simulink model "Example_model"  (R2024b)
settings: Solver=VariableStepAuto  StartTime=0.0  StopTime=60  MaxStep=0.01  RelTol=1e-3
model workspace (MAT data in the model file):
  Sig = Simulink.Signal
  Sig.Dimensions = -1
  Sig.DimensionsMode = 'auto'
  Sig.Complexity = 'auto'
  Sig.SampleTime = -1
  Sig.SamplingMode = 'auto'
  Sig.DataType = 'auto'
  a0 = Simulink.Parameter
  a0.Value = 1
  a0.Complexity = 'real'
  a0.Dimensions = [1 1]
  a0.DataType = 'double'
  a1 = Simulink.Parameter
  a1.Value = 1
  a1.Complexity = 'real'
  a1.Dimensions = [1 1]
  a1.DataType = 'double'
  b0 = Simulink.Parameter
  b0.Value = 1
  b0.Complexity = 'real'
  b0.Dimensions = [1 1]
  b0.DataType = 'double'
  k2 = Simulink.Parameter
  k2.Value = 1
  k2.Complexity = 'real'
  k2.Dimensions = [1 1]
  k2.DataType = 'double'
  k3 = Simulink.Parameter
  k3.Value = 1
  k3.Complexity = 'real'
  k3.Dimensions = [1 1]
  k3.DataType = 'double'
libraries: slpidlib x2
settings Model: Creator=tomkl  LastModifiedBy=tomkl

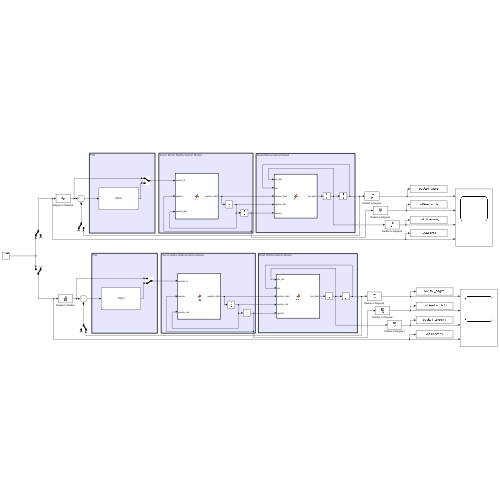
[thumbnail: Simulink's stored preview of the top-level diagram]
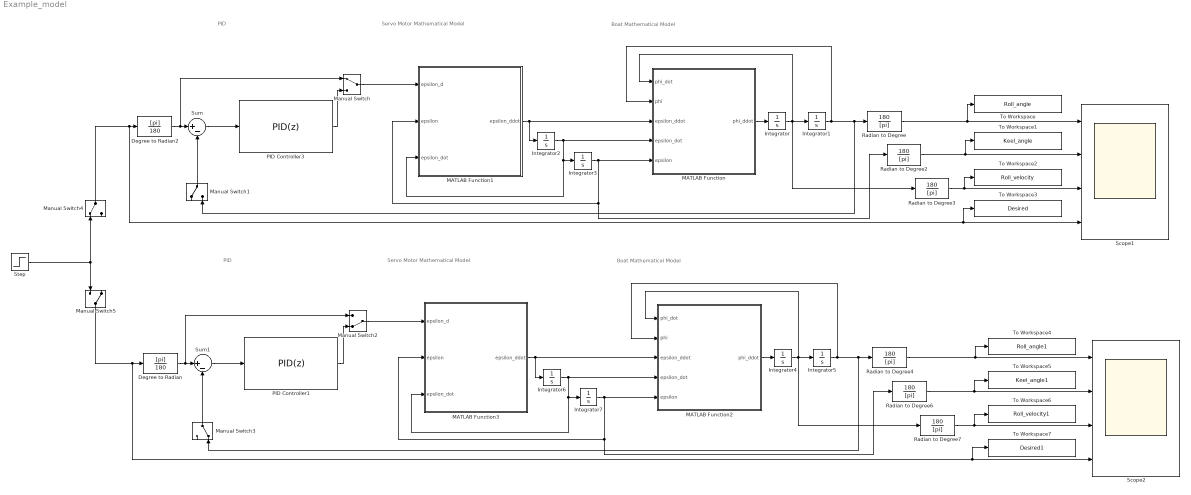
== system Example_model ==
  note: PID
  note: Servo Motor Mathematical Model
  note: Boat Mathematical Model
  note: Servo Motor Mathematical Model
  note: PID
  note: Boat Mathematical Model
  Degree to Radian : TransferFcn  Numerator=[pi]  Denominator=[180]
  Degree to Radian2 : TransferFcn  Numerator=[pi]  Denominator=[180]
  Integrator{,1..7} (8 alike) : Integrator
  MATLAB Function : MATLAB Function  TreatAsAtomicUnit=on
  MATLAB Function1 : MATLAB Function  TreatAsAtomicUnit=on
  MATLAB Function2 : MATLAB Function  TreatAsAtomicUnit=on
  MATLAB Function3 : MATLAB Function  TreatAsAtomicUnit=on
  Manual Switch : ManualSwitch
  Manual Switch1 : ManualSwitch
  Manual Switch2 : ManualSwitch  CurrentSetting=0
  Manual Switch3 : ManualSwitch  CurrentSetting=0
  Manual Switch4 : ManualSwitch
  Manual Switch5 : ManualSwitch  CurrentSetting=0
  PID Controller1 : slpidlib/PID Controller  Controller=PID  Form=Parallel  TimeDomain=Discrete-time  UseExternalTs=off  SampleTime=0.01  IntegratorMethod=Forward Euler  FilterMethod=Forward Euler  ControllerParametersSource=internal  P=0.566467721992697  I=0.110964200934941  UseKiTs=off  D=0.339704255295508  UseExternalDerivativeSource=off  N=1.35164961739647  UseFilter=on  TunerSelectOption=Transfer Function Based (PID Tuner App)  InitialConditionSource=internal  InitialConditionForIntegrator=0  InitialConditionForFilter=0  DifferentiatorICPrevScaledInput=0  ExternalReset=none  TrackingMode=off  Kt=1  LimitOutput=off  SatLimitsSource=internal  UpperSaturationLimit=inf  LowerSaturationLimit=-inf  LinearizeAsGain=on  AntiWindupMode=none  Kb=1  LimitIntegrator=off  UpperIntegratorSaturationLimit=inf  LowerIntegratorSaturationLimit=-inf  POutMin=[]  POutMax=[]  IOutMin=[]  IOutMax=[]  DOutMin=[]  DOutMax=[]  NOutMin=[]  NOutMax=[]  SumOutMin=[]  SumOutMax=[]  SaturationOutMin=[]  SaturationOutMax=[]  PParamMin=[]  PParamMax=[]  IParamMin=[]  IParamMax=[]  DParamMin=[]  DParamMax=[]  NParamMin=[]  NParamMax=[]  KbParamMin=[]  KbParamMax=[]  KtParamMin=[]  KtParamMax=[]  KbOutMin=[]  KbOutMax=[]  KtOutMin=[]  KtOutMax=[]  IntegratorOutMin=[]  IntegratorOutMax=[]  FilterOutMin=[]  FilterOutMax=[]  SumI1OutMin=[]  SumI1OutMax=[]  SumI2OutMin=[]  SumI2OutMax=[]  SumI3OutMin=[]  SumI3OutMax=[]  SumI4OutMin=[]  SumI4OutMax=[]  SumDOutMin=[]  SumDOutMax=[]  DifferentiatorOutMin=[]  DifferentiatorOutMax=[]  FilterDiffOutCoefMin=[]  FilterDiffOutCoefMax=[]  ReciprocalOutMin=[]  ReciprocalOutMax=[]  SumDenOutMin=[]  SumDenOutMax=[]  SumNumOutMin=[]  SumNumOutMax=[]  DivideOutMin=[]  DivideOutMax=[]  UdiffTsProdOutMin=[]  UdiffTsProdOutMax=[]  NTsProdOutMin=[]  NTsProdOutMax=[]  UintegralTsProdOutMin=[]  UintegralTsProdOutMax=[]  UngainTsProdOutMin=[]  UngainTsProdOutMax=[]  ClampingZeroOutDataTypeStr=Inherit: Inherit via back propagation  ClampingZeroOutMin=[]  ClampingZeroOutMax=[]  FilterDenConstantOutDataTypeStr=Inherit: Inherit via back propagation  FilterDenConstantOutMin=[]  FilterDenConstantOutMax=[]  PCopyOutDataTypeStr=Inherit: Inherit via back propagation  PCopyOutMin=[]  PCopyOutMax=[]  NCopyOutDataTypeStr=Inherit: Inherit via back propagation  NCopyOutMin=[]  NCopyOutMax=[]  IntegratorContinuousStateAttributes=''  IntegratorStateMustResolveToSignalObject=off  IntegratorRTWStateStorageClass=Auto  FilterContinuousStateAttributes=''  FilterStateMustResolveToSignalObject=off  FilterRTWStateStorageClass=Auto  ParallelPVariant=InternalParameters  IdealPVariant=Disabled  IVariant=InternalParameters  DVariant=InternalParameters  IntegratorVariant=Discrete  SatVariant=Disabled  AWVariant=Passthrough  PCopyVariant=Disabled  TRVariant=Disabled  FdbkBlocksVariant=Forward  IdealPFdbkVariant=Disabled  SatFdbkVariant=Disabled  DerivativeFilterVariant=ForwardEulerFilter  NVariant=InternalParameters  NCopyVariant=Disabled  FilterICVariant=InternalICsFilter  IntegratorICVariant=InternalICs  ExternalResetVariant=Disabled  TRSumVariant=Passthrough  SumFdbkVariant=Disabled  SumVariant=Sum_PID  TsampFilterVariant=InternalTs  TsampNgainVariant=Passthrough  TsampIntegralVariant=Disabled_SignalSpec  ExternalSaturationOutDataTypeStr=Inherit: Same as second input  DerivativeSourceVariant=ErrorSignal  PreIntVariant=InternalPreInt
  PID Controller3 : slpidlib/PID Controller  Controller=PID  Form=Parallel  TimeDomain=Discrete-time  UseExternalTs=off  SampleTime=0.01  IntegratorMethod=Forward Euler  FilterMethod=Forward Euler  ControllerParametersSource=internal  P=0.566467721992697  I=0.110964200934941  UseKiTs=off  D=0.339704255295508  UseExternalDerivativeSource=off  N=1.35164961739647  UseFilter=on  TunerSelectOption=Transfer Function Based (PID Tuner App)  InitialConditionSource=internal  InitialConditionForIntegrator=0  InitialConditionForFilter=0  DifferentiatorICPrevScaledInput=0  ExternalReset=none  TrackingMode=off  Kt=1  LimitOutput=off  SatLimitsSource=internal  UpperSaturationLimit=inf  LowerSaturationLimit=-inf  LinearizeAsGain=on  AntiWindupMode=none  Kb=1  LimitIntegrator=off  UpperIntegratorSaturationLimit=inf  LowerIntegratorSaturationLimit=-inf  POutMin=[]  POutMax=[]  IOutMin=[]  IOutMax=[]  DOutMin=[]  DOutMax=[]  NOutMin=[]  NOutMax=[]  SumOutMin=[]  SumOutMax=[]  SaturationOutMin=[]  SaturationOutMax=[]  PParamMin=[]  PParamMax=[]  IParamMin=[]  IParamMax=[]  DParamMin=[]  DParamMax=[]  NParamMin=[]  NParamMax=[]  KbParamMin=[]  KbParamMax=[]  KtParamMin=[]  KtParamMax=[]  KbOutMin=[]  KbOutMax=[]  KtOutMin=[]  KtOutMax=[]  IntegratorOutMin=[]  IntegratorOutMax=[]  FilterOutMin=[]  FilterOutMax=[]  SumI1OutMin=[]  SumI1OutMax=[]  SumI2OutMin=[]  SumI2OutMax=[]  SumI3OutMin=[]  SumI3OutMax=[]  SumI4OutMin=[]  SumI4OutMax=[]  SumDOutMin=[]  SumDOutMax=[]  DifferentiatorOutMin=[]  DifferentiatorOutMax=[]  FilterDiffOutCoefMin=[]  FilterDiffOutCoefMax=[]  ReciprocalOutMin=[]  ReciprocalOutMax=[]  SumDenOutMin=[]  SumDenOutMax=[]  SumNumOutMin=[]  SumNumOutMax=[]  DivideOutMin=[]  DivideOutMax=[]  UdiffTsProdOutMin=[]  UdiffTsProdOutMax=[]  NTsProdOutMin=[]  NTsProdOutMax=[]  UintegralTsProdOutMin=[]  UintegralTsProdOutMax=[]  UngainTsProdOutMin=[]  UngainTsProdOutMax=[]  ClampingZeroOutDataTypeStr=Inherit: Inherit via back propagation  ClampingZeroOutMin=[]  ClampingZeroOutMax=[]  FilterDenConstantOutDataTypeStr=Inherit: Inherit via back propagation  FilterDenConstantOutMin=[]  FilterDenConstantOutMax=[]  PCopyOutDataTypeStr=Inherit: Inherit via back propagation  PCopyOutMin=[]  PCopyOutMax=[]  NCopyOutDataTypeStr=Inherit: Inherit via back propagation  NCopyOutMin=[]  NCopyOutMax=[]  IntegratorContinuousStateAttributes=''  IntegratorStateMustResolveToSignalObject=off  IntegratorRTWStateStorageClass=Auto  FilterContinuousStateAttributes=''  FilterStateMustResolveToSignalObject=off  FilterRTWStateStorageClass=Auto  ParallelPVariant=InternalParameters  IdealPVariant=Disabled  IVariant=InternalParameters  DVariant=InternalParameters  IntegratorVariant=Discrete  SatVariant=Disabled  AWVariant=Passthrough  PCopyVariant=Disabled  TRVariant=Disabled  FdbkBlocksVariant=Forward  IdealPFdbkVariant=Disabled  SatFdbkVariant=Disabled  DerivativeFilterVariant=ForwardEulerFilter  NVariant=InternalParameters  NCopyVariant=Disabled  FilterICVariant=InternalICsFilter  IntegratorICVariant=InternalICs  ExternalResetVariant=Disabled  TRSumVariant=Passthrough  SumFdbkVariant=Disabled  SumVariant=Sum_PID  TsampFilterVariant=InternalTs  TsampNgainVariant=Passthrough  TsampIntegralVariant=Disabled_SignalSpec  ExternalSaturationOutDataTypeStr=Inherit: Same as second input  DerivativeSourceVariant=ErrorSignal  PreIntVariant=InternalPreInt
  Radian to Degree{,2..4,6..7} (6 alike) : TransferFcn  Numerator=[180]  Denominator=[pi]
  Scope1 : Scope  NumInputPorts=4
  Scope2 : Scope  NumInputPorts=4
  Step : Step  SampleTime=0
  Sum : Sum  Inputs=|+-
  Sum1 : Sum  Inputs=|+-
  To Workspace : ToWorkspace  VariableName=Roll_angle  SaveFormat=Timeseries  SampleTime=-1
  To Workspace1 : ToWorkspace  VariableName=Keel_angle  SaveFormat=Timeseries  SampleTime=-1
  To Workspace2 : ToWorkspace  VariableName=Roll_velocity  SaveFormat=Timeseries  SampleTime=-1
  To Workspace3 : ToWorkspace  VariableName=Desired  SaveFormat=Timeseries  SampleTime=-1
  To Workspace4 : ToWorkspace  VariableName=Roll_angle1  SaveFormat=Timeseries  SampleTime=-1
  To Workspace5 : ToWorkspace  VariableName=Keel_angle1  SaveFormat=Timeseries  SampleTime=-1
  To Workspace6 : ToWorkspace  VariableName=Roll_velocity1  SaveFormat=Timeseries  SampleTime=-1
  To Workspace7 : ToWorkspace  VariableName=Desired1  SaveFormat=Timeseries  SampleTime=-1
  wires:
  MATLAB Function/1(phi_ddot) -> Integrator/1
  Integrator/1 -> Radian to Degree3/1, MATLAB Function/1(phi_dot), Integrator1/1
  Integrator1/1 -> Manual Switch1/2, Radian to Degree/1, MATLAB Function/2(phi)
  Integrator3/1 -> Radian to Degree2/1, MATLAB Function1/2(epsilon), MATLAB Function/5(epsilon)
  Integrator2/1 -> MATLAB Function/4(epsilon_dot), MATLAB Function1/3(epsilon_dot), Integrator3/1
  MATLAB Function1/1(epsilon_ddot) -> Integrator2/1, MATLAB Function/3(epsilon_ddot)
  Radian to Degree/1 -> Scope1/1, To Workspace/1
  Sum/1 -> PID Controller3/1
  Manual Switch/1 -> MATLAB Function1/1(epsilon_d)
  PID Controller3/1 -> Manual Switch/2
  Manual Switch1/1 -> Sum/2
  Degree to Radian2/1 -> Manual Switch/1, Sum/1
  Radian to Degree2/1 -> To Workspace1/1, Scope1/2
  Radian to Degree3/1 -> Scope1/3, To Workspace2/1
  Radian to Degree7/1 -> To Workspace6/1, Scope2/3
  MATLAB Function3/1(epsilon_ddot) -> Integrator6/1, MATLAB Function2/3(epsilon_ddot)
  Integrator5/1 -> Radian to Degree4/1, Manual Switch3/2, MATLAB Function2/2(phi)
  Radian to Degree4/1 -> To Workspace4/1, Scope2/1
  Radian to Degree6/1 -> Scope2/2, To Workspace5/1
  PID Controller1/1 -> Manual Switch2/2
  Degree to Radian/1 -> Manual Switch2/1, Sum1/1
  Integrator6/1 -> MATLAB Function2/4(epsilon_dot), MATLAB Function3/3(epsilon_dot), Integrator7/1
  Manual Switch2/1 -> MATLAB Function3/1(epsilon_d)
  Integrator4/1 -> Radian to Degree7/1, MATLAB Function2/1(phi_dot), Integrator5/1
  Manual Switch3/1 -> Sum1/2
  Sum1/1 -> PID Controller1/1
  MATLAB Function2/1(phi_ddot) -> Integrator4/1
  Integrator7/1 -> Radian to Degree6/1, MATLAB Function3/2(epsilon), MATLAB Function2/5(epsilon)
  Manual Switch4/1 -> Scope1/4, To Workspace3/1, Degree to Radian2/1
  Manual Switch5/1 -> Scope2/4, To Workspace7/1, Degree to Radian/1
  Step/1 -> Manual Switch4/1, Manual Switch5/1

== matlab function Example_model/MATLAB Function1 ==
  data: epsilon_d input; epsilon input; epsilon_dot input; epsilon_ddot output
function epsilon_ddot=fcn(epsilon_d,epsilon,epsilon_dot)

%defining variables
u=epsilon_d;                       %input value
k_t = 100;                         %Motor torque constant [Nm/A]
k_pm = 1250;                       %Motor controller proportional gain
J_km = 20*10^3;                    %Motor inertia coefficient [kgm^2] 
R_a = 1;                           %Motor armature resistance [ohm]
k_b = 375;                         %Motor Back-Emf constant [Vs/rad]
k_dm = 0.3;                        %Motor controller derivative gain
B_km = 100;                        %Motor damping coefficient [Nms/rad]
alpha_1 = (-k_t*k_pm)/(J_km*R_a);
alpha_2 = (-k_t*(k_b+k_dm)-R_a*B_km)/(J_km*R_a);
Beta = (k_t*k_pm)/(J_km*R_a);

%J_km, B_km are in both function block, care for it while changing values

%defining funciton
epsilon_ddot=alpha_1*epsilon+alpha_2*epsilon_dot+Beta*u;

== matlab function Example_model/MATLAB Function ==
  data: phi_dot input; phi input; epsilon_ddot input; epsilon_dot input; phi_ddot output; epsilon input
function phi_ddot=fcn(phi_dot, phi, epsilon_ddot, epsilon_dot, epsilon)

%defining contants
rho = 1025;           %Density of sea water [kg/m^3]
g = 9.81;             %Gravity [m/s^2]

I_x = 125000;         %Roll moment of inertia of the vessel [kgm^2]
delta_I_x = 31250;    %Hydrodynamic added mass coefficient  [kgm^2]
nabla = 20000/rho;        %Volume displacement of the ship [kg]
GMm_bar = 1.06;       %Mean metacentric height [m]
K_dphi = 1*10^5;      %Linear positive drag coefficient in roll [kgm^2/s]
K_dphidphi = 0.5*10^5;%Non-linear positive drag coefficient in roll [kgm^2]

m_k = 150;            %Mass of the keel system [kg]
nabla_k = 6;          %Volume of the keel system [m^3]
z_k = 1.4;            %Distance between the vessels center of mass and the hinge point of the keel [m]                 
L_k = 2;              %Distance between the hinge point to the mass/buoancy center of keel system [m]

J_km = 20*10^3;       %Motor intertia coefficient [kgm^2]
B_km = 100;           %Motor damping coefficient [NMs/rad]

m_d = 300;            %Mass of the load in the vessel frame [kgs]
y_d = 0.5;            %Lateral position of the load of mass in the vessel frame [m]
z_d = 2.5;            %Vertical position of the load of mass from the center of mass of the vessel [m]


K_phi3 = 3;           %Not specified
K_k = 1000;           %K_dphi;
K_kk = 500;           %K_dphidphi;
delta_m_k = 6150;        %Added mass coefficient of the keel - not speficied

%defining function
phi_ddot = ( ...
    -K_dphi*phi_dot ...
    -K_dphidphi*phi_dot*abs(phi_dot) ...
    -rho*g*nabla*GMm_bar*phi ...
    -K_phi3*phi^3 ...
    -(m_k-rho*nabla_k)*g*(z_k*sin(phi)+L_k*sin(epsilon+phi)) ...
    -K_k*(epsilon_dot+phi_dot) -K_kk*(epsilon_dot+phi_dot)*abs(epsilon_dot-phi_dot) ...
    -J_km*epsilon_ddot-B_km*epsilon_dot ...
    +m_d*g*(z_d*sin(phi)+y_d*cos(phi))...
    -delta_m_k*epsilon_ddot)/(I_x+delta_I_x+delta_m_k);

== matlab function Example_model/MATLAB Function2 ==
  data: phi_dot input; phi input; epsilon_ddot input; epsilon_dot input; phi_ddot output; epsilon input
function phi_ddot=fcn(phi_dot, phi, epsilon_ddot, epsilon_dot, epsilon)

%defining contants
rhi = 1025;           %Density of sea water [kg/m^3]
g = 9.81;             %Gravity [m/s^2]

I_x = 125000;         %Roll moment of inertia of the vessel [kgm^2]
delta_I_x = 31250;    %Hydrodynamic added mass coefficient  [kgm^2]
nabla = 20000/rhi;        %Volume displacement of the ship [kg]
GMm_bar = 1.06;       %Mean metacentric height [m]
K_dphi = 1*10^5;      %Linear positive drag coefficient in roll [kgm^2/s]
K_dphidphi = 0.5*10^5;%Non-linear positive drag coefficient in roll [kgm^2]

m_k = 150;            %Mass of the keel system [kg]
nabla_k = 6;          %Volume of the keel system [m^3]
z_k = 1.4;            %Distance between the vessels center of mass and the hinge point of the keel [m]                 
L_k = 2;              %Distance between the hinge point to the mass/buoancy center of keel system [m]

J_km = 20*10^3;       %Motor intertia coefficient [kgm^2]
B_km = 100;           %Motor damping coefficient [NMs/rad]

m_d = 300;            %Mass of the load in the vessel frame [kgs]
y_d = 0.5;            %Lateral position of the load of mass in the vessel frame [m]
z_d = 2.5;            %Vertical position of the load of mass from the center of mass of the vessel [m]


K_phi3 = 3;           %Not specified
K_k = 1000;           %K_dphi;
K_kk = 500;           %K_dphidphi;
delta_m_k = 6150;        %Added mass coefficient of the keel - not speficied

%defining function
phi_ddot = ( ...
    -K_dphi*phi_dot ... 
    -rhi*g*nabla*GMm_bar*phi ...
    -(m_k-rhi*nabla_k)*g*(z_k*(phi)+L_k*(epsilon+phi)) ...
    -K_k*(epsilon_dot+phi_dot)...
    -J_km*epsilon_ddot-B_km*epsilon_dot ...
    -delta_m_k*epsilon_ddot)/(I_x+delta_I_x+delta_m_k);

== matlab function Example_model/MATLAB Function3 ==
  data: epsilon_d input; epsilon input; epsilon_dot input; epsilon_ddot output
function epsilon_ddot=fcn(epsilon_d,epsilon,epsilon_dot)

%defining variables
u=epsilon_d;                       %input value
k_t = 100;                         %Motor torque constant [Nm/A]
k_pm = 1250;                       %Motor controller proportional gain
J_km = 20*10^3;                    %Motor inertia coefficient [kgm^2] 
R_a = 1;                           %Motor armature resistance [ohm]
k_b = 375;                         %Motor Back-Emf constant [Vs/rad]
k_dm = 0.3;                        %Motor controller derivative gain
B_km = 100;                        %Motor damping coefficient [Nms/rad]
alpha_1 = (-k_t*k_pm)/(J_km*R_a);
alpha_2 = (-k_t*(k_b+k_dm)-R_a*B_km)/(J_km*R_a);
Beta = (k_t*k_pm)/(J_km*R_a);

%J_km, B_km are in both function block, care for it while changing values

%defining funciton
epsilon_ddot=alpha_1*epsilon+alpha_2*epsilon_dot+Beta*u;
